simulink model "lab3d"  (R2022b)
settings: Solver=FixedStepAuto  StartTime=0.0  StopTime=1.0  FixedStep=1/1024  RelTol=1e-3
values from neighbouring files (symbols this model uses):
  amp = i    [lab3a.m]    (also in lab3a_script.m = db2mag(cur_pow); lab3bscript.m)
  f = f*10    (= 50)    [lab3a_script.m]
settings Model: Creator=simja  LastModifiedBy=simja
settings DataIOCC: ReturnWorkspaceOutputs=off

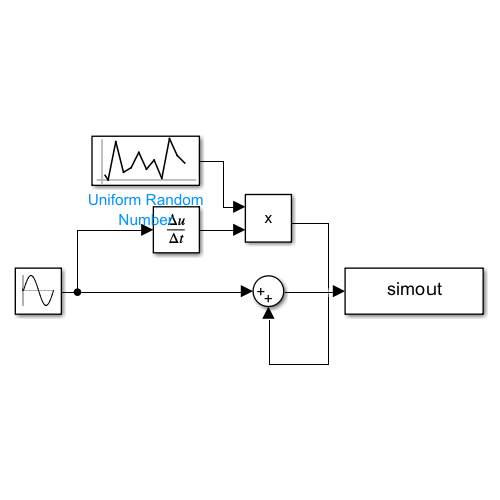
[thumbnail: Simulink's stored preview of the top-level diagram]
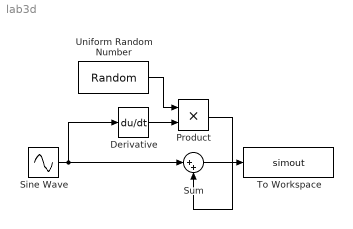
== system lab3d ==
  Derivative : Derivative
  Product : Product
  Sine Wave : Sin  Amplitude=amp  Frequency=2*f*pi  SampleTime=0
  Sum : Sum  Inputs=|++
  To Workspace : ToWorkspace  VariableName=simout  SaveFormat=Structure With Time  SampleTime=-1
  Uniform Random Number : UniformRandomNumber  Minimum=-0.1/1024  Maximum=0.1/1024  SampleTime=0
  wires:
  Sine Wave/1 -> Sum/1, Derivative/1
  Derivative/1 -> Product/2
  Uniform Random Number/1 -> Product/1
  Product/1 -> Sum/2
  Sum/1 -> To Workspace/1
